simulink model "MaglevLinear"  (R2018a)
settings: Solver=VariableStepAuto  StartTime=0.0  StopTime=10.0  RelTol=1e-3
settings Model: Creator=saad  LastModifiedBy=saad

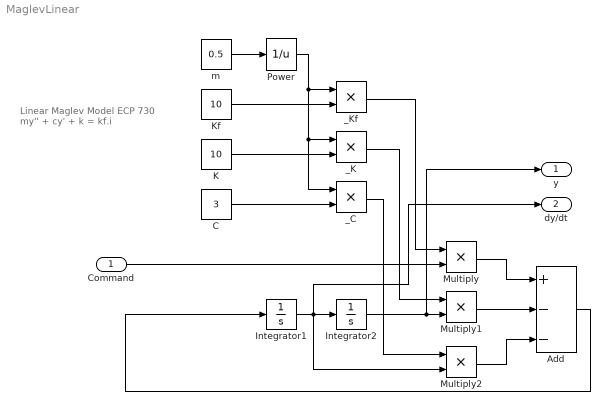
== system MaglevLinear ==
  note: Linear Maglev Model
      | ECP 730
      |
      | my'' + cy' + k = kf.i
  Command : Inport
  Add : Sum  Inputs=+--
  C : Constant  Value=3
  Integrator1 : Integrator
  Integrator2 : Integrator
  K : Constant  Value=10
  Kf : Constant  Value=10
  Multiply : Product
  Multiply1 : Product
  Multiply2 : Product
  Power : Math  Operator=reciprocal  SaturateOnIntegerOverflow=on
  _C : Product
  _K : Product
  _Kf : Product
  m : Constant  Value=0.5
  y : Outport
  dy/dt : Outport  Port=2
  wires:
  m/1 -> Power/1
  C/1 -> _C/2
  K/1 -> _K/2
  Kf/1 -> _Kf/2
  Power/1 -> _Kf/1, _K/1, _C/1
  Command/1 -> Multiply/2
  _Kf/1 -> Multiply/1
  Add/1 -> Integrator1/1
  Integrator1/1 -> dy/dt/1, Multiply2/2, Integrator2/1
  Integrator2/1 -> y/1, Multiply1/2
  _K/1 -> Multiply1/1
  _C/1 -> Multiply2/1
  Multiply/1 -> Add/1
  Multiply1/1 -> Add/2
  Multiply2/1 -> Add/3
